simulink library "BEML_EMU_TractionInput_Lib"  (R2019b)
settings: Solver=VariableStepAuto  StartTime=0.0  StopTime=10.0  RelTol=1e-3
undefined symbols (not defined in the file): Bogie, BogieIsolationStatus, BogieSupportedMass, ContactorsFailure, DynamicBrakeForceVariation, Dynamics, ElectricalSystem, ForwardTW, HeavyWheelSlide, HeavyWheelSlip, NoEmergencyBrakeActiveTW, PowerAvailable, ReverseTW, TCMS, TCMSDynamicBrakingInhibit, TCMSEDBrakingCmd, TCMSTractionCmd, TCMSTractionInhibit, TCUPower, TractionActiveTW, TractionAuthorisation, TractionCutoff, TractionForceVariation, TractionSampleTime, TractiveLosses, VCBState, Velocity, WheelSlide, WheelSlip, WheelSpeed
libraries: simulink x4
settings Model: Creator=rleighton  LastModifiedBy=hinganes
settings DebuggingCC: ArithmeticOperatorsInVariantConditions=warning
settings SFSimCC: SimUseLocalCustomCode=off  CustomCodeUndefinedFunction=UseInterfaceOnly
settings RTWCC: RTWUseLocalCustomCode=off

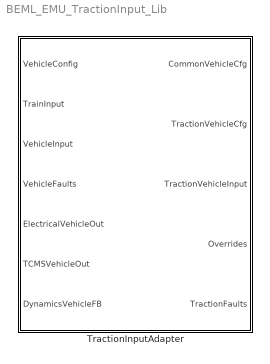
== system BEML_EMU_TractionInput_Lib ==
  TractionInputAdapter : Subsystem  TreatAsAtomicUnit=on  SystemSampleTime=TractionSampleTime

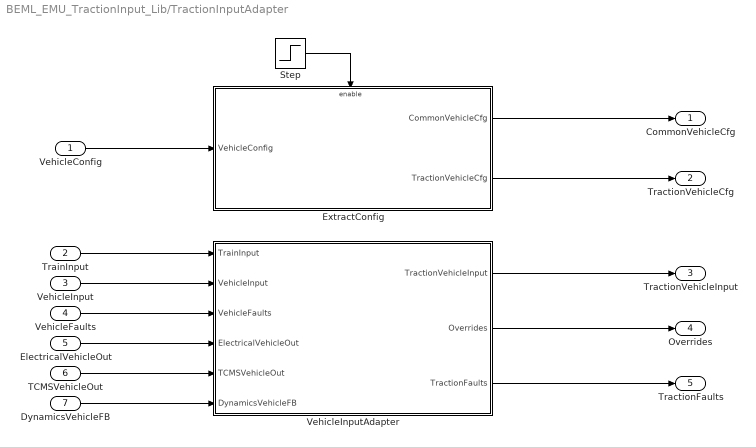
== system BEML_EMU_TractionInput_Lib/TractionInputAdapter ==
  VehicleConfig : Inport
  TrainInput : Inport  Port=2
  VehicleInput : Inport  Port=3
  VehicleFaults : Inport  Port=4
  ElectricalVehicleOut : Inport  Port=5
  TCMSVehicleOut : Inport  Port=6
  DynamicsVehicleFB : Inport  Port=7
  ExtractConfig : Subsystem
  Step : Step  Before=1  After=0
  VehicleInputAdapter : Subsystem
  CommonVehicleCfg : Outport  VectorParamsAs1DForOutWhenUnconnected=off
  TractionVehicleCfg : Outport  Port=2  VectorParamsAs1DForOutWhenUnconnected=off
  TractionVehicleInput : Outport  Port=3  VectorParamsAs1DForOutWhenUnconnected=off
  Overrides : Outport  Port=4  VectorParamsAs1DForOutWhenUnconnected=off
  TractionFaults : Outport  Port=5  VectorParamsAs1DForOutWhenUnconnected=off
  wires:
  TCMSVehicleOut/1 -> VehicleInputAdapter/5(TCMSVehicleOut)
  VehicleInputAdapter/3(TractionFaults) -> TractionFaults/1
  VehicleInputAdapter/2(Overrides) -> Overrides/1
  VehicleInputAdapter/1(TractionVehicleInput) -> TractionVehicleInput/1
  VehicleFaults/1 -> VehicleInputAdapter/3(VehicleFaults)
  Step/1 -> ExtractConfig/Enable
  ExtractConfig/2(TractionVehicleCfg) -> TractionVehicleCfg/1
  ExtractConfig/1(CommonVehicleCfg) -> CommonVehicleCfg/1
  VehicleConfig/1 -> ExtractConfig/1(VehicleConfig)
  DynamicsVehicleFB/1 -> VehicleInputAdapter/6(DynamicsVehicleFB)
  ElectricalVehicleOut/1 -> VehicleInputAdapter/4(ElectricalVehicleOut)
  VehicleInput/1 -> VehicleInputAdapter/2(VehicleInput)
  TrainInput/1 -> VehicleInputAdapter/1(TrainInput)

== system BEML_EMU_TractionInput_Lib/TractionInputAdapter/ExtractConfig ==
  VehicleConfig : Inport
  Enable : EnablePort
  ExtractConfig : Subsystem
  CommonVehicleCfg : Outport  VectorParamsAs1DForOutWhenUnconnected=off
  TractionVehicleCfg : Outport  Port=2  VectorParamsAs1DForOutWhenUnconnected=off
  wires:
  VehicleConfig/1 -> ExtractConfig/1(VehicleConfig)
  ExtractConfig/1(CommonVehicleConfig) -> CommonVehicleCfg/1
  ExtractConfig/2(TractionVehicleConfig) -> TractionVehicleCfg/1

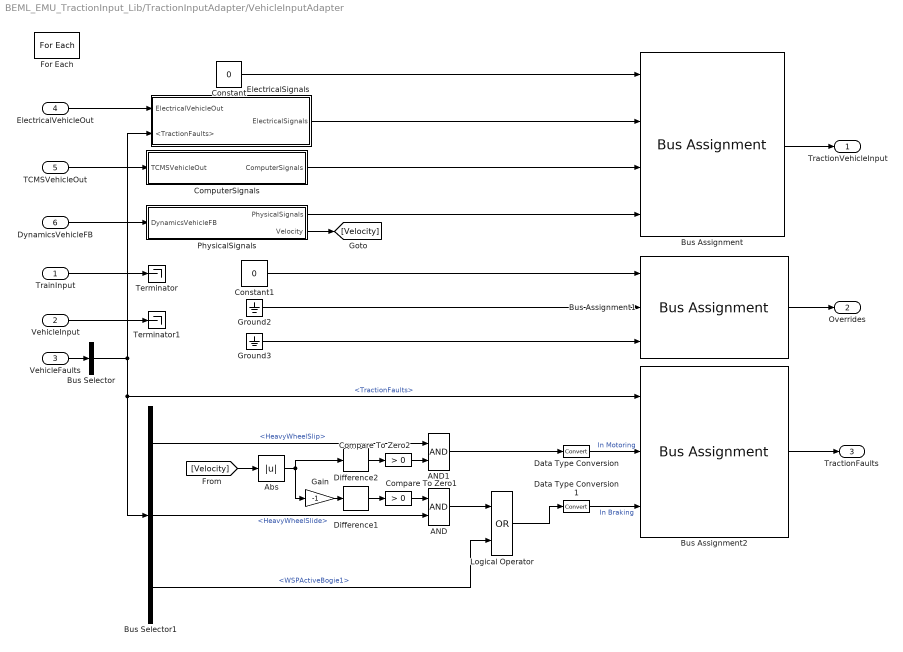
== system BEML_EMU_TractionInput_Lib/TractionInputAdapter/VehicleInputAdapter ==
  TrainInput : Inport
  VehicleInput : Inport  Port=2
  VehicleFaults : Inport  Port=3  Partition=on  PartitionDimension=1  PartitionWidth=1  PartitionOffset=0
  ElectricalVehicleOut : Inport  Port=4  Partition=on  PartitionDimension=1  PartitionWidth=1  PartitionOffset=0
  TCMSVehicleOut : Inport  Port=5  Partition=on  PartitionDimension=1  PartitionWidth=1  PartitionOffset=0
  DynamicsVehicleFB : Inport  Port=6  Partition=on  PartitionDimension=1  PartitionWidth=1  PartitionOffset=0
  AND : Logic  AllPortsSameDT=off  OutDataTypeStr=boolean
  AND1 : Logic  AllPortsSameDT=off  OutDataTypeStr=boolean
  Abs : Abs
  Bus Assignment : BusAssignment  AssignedSignals=ElectricalSystem,TCMS,Dynamics
  Bus Assignment1 : BusAssignment  AssignedSignals=TractionForceVariation,DynamicBrakeForceVariation
  Bus Assignment2 : BusAssignment  AssignedSignals=HeavyWheelSlip,HeavyWheelSlide
  Bus Selector : BusSelector  OutputSignals=TractionFaults
  Bus Selector1 : BusSelector  OutputSignals=HeavyWheelSlip,HeavyWheelSlide,WSPActiveBogie1
  Compare To Zero1 : simulink/Logic and Bit Operations/Compare To Zero  relop=>  OutDataTypeStr=boolean
  Compare To Zero2 : simulink/Logic and Bit Operations/Compare To Zero  relop=>  OutDataTypeStr=boolean
  ComputerSignals : Subsystem
  Constant : Constant  Value=0  OutDataTypeStr=Bus: BD_TractionSystem_In_Vehicle
  Constant1 : Constant  Value=0  OutDataTypeStr=Bus: BD_TractionSystem_In_Overrides
  Data Type Conversion : DataTypeConversion
  Data Type Conversion1 : DataTypeConversion
  Difference1 : simulink/Discrete/Difference  ICPrevInput=0.0  OutMin=[]  OutMax=[]  OutDataType=fixdt(1, 16)  OutScaling=2^-10  DoSatur=off
  Difference2 : simulink/Discrete/Difference  ICPrevInput=0.0  OutMin=[]  OutMax=[]  OutDataType=fixdt(1, 16)  OutScaling=2^-10  DoSatur=off
  ElectricalSignals : Subsystem
  For Each : ForEach  DisableCoverage=on
  Gain : Gain  Gain=-1
  Ground2 : Ground
  Ground3 : Ground
  Logical Operator : Logic  Operator=OR  AllPortsSameDT=off  OutDataTypeStr=boolean
  PhysicalSignals : Subsystem
  Terminator : Terminator
  Terminator1 : Terminator
  TractionVehicleInput : Outport  ConcatenationDimension=1  VectorParamsAs1DForOutWhenUnconnected=off
  Overrides : Outport  Port=2  ConcatenationDimension=1  VectorParamsAs1DForOutWhenUnconnected=off
  TractionFaults : Outport  Port=3  ConcatenationDimension=1  VectorParamsAs1DForOutWhenUnconnected=off
  wires:
  Logical Operator/1 -> Data Type Conversion1/1
  Bus Selector1/3 -> Logical Operator/2  "<WSPActiveBogie1>"
  VehicleInput/1 -> Terminator1/1
  Abs/1 -> Gain/1, Difference2/1
  Data Type Conversion1/1 -> Bus Assignment2/3  "In Braking"
  Data Type Conversion/1 -> Bus Assignment2/2  "In Motoring"
  AND/1 -> Logical Operator/1
  AND1/1 -> Data Type Conversion/1
  Compare To Zero2/1 -> AND1/2
  Difference2/1 -> Compare To Zero2/1
  [Velocity] -> Abs/1
  Bus Selector1/1 -> AND1/1  "<HeavyWheelSlip>"
  Bus Selector1/2 -> AND/2  "<HeavyWheelSlide>"
  PhysicalSignals/2(Velocity) -> [Velocity]
  Gain/1 -> Difference1/1
  Difference1/1 -> Compare To Zero1/1
  Compare To Zero1/1 -> AND/1
  Bus Assignment2/1 -> TractionFaults/1
  TCMSVehicleOut/1 -> ComputerSignals/1(TCMSVehicleOut)
  DynamicsVehicleFB/1 -> PhysicalSignals/1(DynamicsVehicleFB)
  ComputerSignals/1(ComputerSignals) -> Bus Assignment/3
  ElectricalSignals/1(ElectricalSignals) -> Bus Assignment/2
  Bus Selector/1 -> ElectricalSignals/2(<TractionFaults>), Bus Selector1/1, Bus Assignment2/1  "<TractionFaults>"
  Bus Assignment1/1 -> Overrides/1
  Ground2/1 -> Bus Assignment1/2
  Ground3/1 -> Bus Assignment1/3
  Constant1/1 -> Bus Assignment1/1
  Bus Assignment/1 -> TractionVehicleInput/1
  Constant/1 -> Bus Assignment/1
  ElectricalVehicleOut/1 -> ElectricalSignals/1(ElectricalVehicleOut)
  VehicleFaults/1 -> Bus Selector/1
  TrainInput/1 -> Terminator/1
  PhysicalSignals/1(PhysicalSignals) -> Bus Assignment/4

== system BEML_EMU_TractionInput_Lib/TractionInputAdapter/ExtractConfig/ExtractConfig ==
  VehicleConfig : Inport  Partition=on  PartitionDimension=1  PartitionWidth=1  PartitionOffset=0  BusOutputAsStruct=on
  Bus Selector : BusSelector  OutputSignals=Common,Traction
  For Each : ForEach  DisableCoverage=on
  CommonVehicleConfig : Outport  ConcatenationDimension=1  VectorParamsAs1DForOutWhenUnconnected=off
  TractionVehicleConfig : Outport  Port=2  ConcatenationDimension=1  VectorParamsAs1DForOutWhenUnconnected=off
  wires:
  Bus Selector/2 -> TractionVehicleConfig/1  "<Traction>"
  Bus Selector/1 -> CommonVehicleConfig/1  "<Common>"
  VehicleConfig/1 -> Bus Selector/1

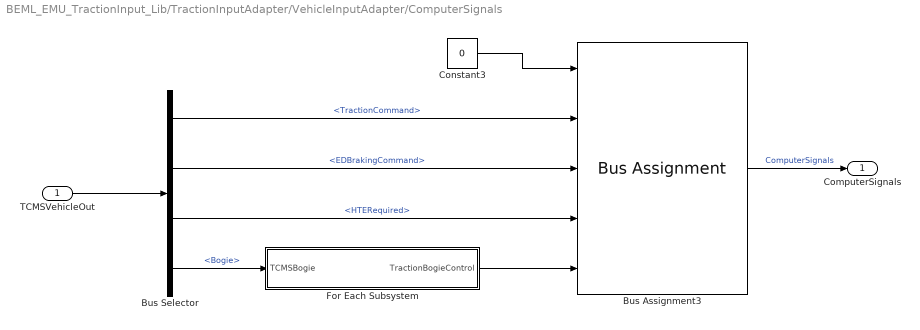
== system BEML_EMU_TractionInput_Lib/TractionInputAdapter/VehicleInputAdapter/ComputerSignals ==
  TCMSVehicleOut : Inport
  Bus Assignment3 : BusAssignment  AssignedSignals=TCMSTractionCmd,TCMSEDBrakingCmd,TractiveLosses,Bogie
  Bus Selector : BusSelector  OutputSignals=Control.TractionSBraking.TractionCommand,Control.TractionSBraking.EDBrakingCommand,Control.TractionSBraking.HTERequired,Control.TractionSBraking.Bogie
  Constant3 : Constant  Value=0  OutDataTypeStr=Bus: BD_TractionSystem_In_Vehicle_TCMS
  For Each Subsystem : Subsystem  TreatAsAtomicUnit=on
  ComputerSignals : Outport
  wires:
  Bus Selector/3 -> Bus Assignment3/4  "<HTERequired>"
  For Each Subsystem/1(TractionBogieControl) -> Bus Assignment3/5
  Bus Selector/2 -> Bus Assignment3/3  "<EDBrakingCommand>"
  Bus Selector/1 -> Bus Assignment3/2  "<TractionCommand>"
  Bus Selector/4 -> For Each Subsystem/1(TCMSBogie)  "<Bogie>"
  Constant3/1 -> Bus Assignment3/1
  Bus Assignment3/1 -> ComputerSignals/1  "ComputerSignals"
  TCMSVehicleOut/1 -> Bus Selector/1

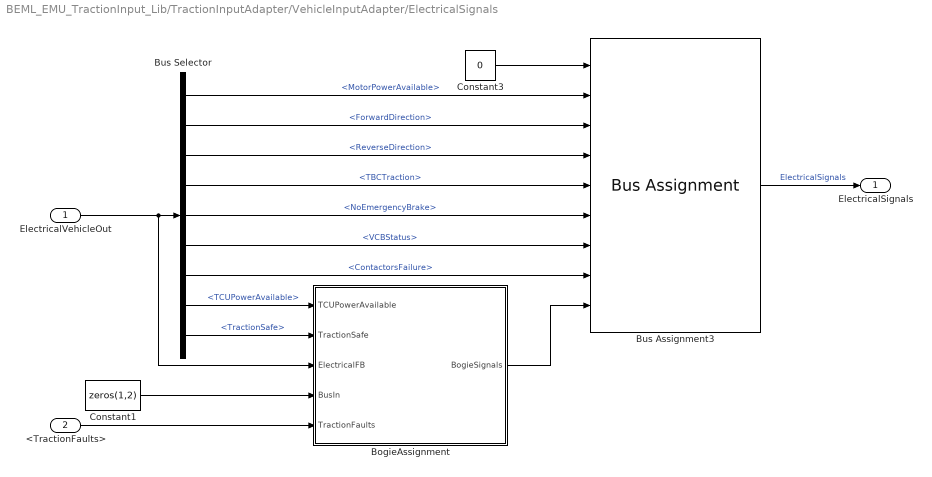
== system BEML_EMU_TractionInput_Lib/TractionInputAdapter/VehicleInputAdapter/ElectricalSignals ==
  ElectricalVehicleOut : Inport
  <TractionFaults> : Inport  Port=2
  BogieAssignment : Subsystem  TreatAsAtomicUnit=on
  Bus Assignment3 : BusAssignment  AssignedSignals=PowerAvailable,ForwardTW,ReverseTW,TractionActiveTW,NoEmergencyBrakeActiveTW,VCBState,ContactorsFailure,Bogie
  Bus Selector : BusSelector  OutputSignals=Traction.MotorPowerAvailable,Traction.ForwardDirection,Traction.ReverseDirection,Traction.TBCTraction,Traction.NoEmergencyBrake,Traction.VCBStatus,Traction.ContactorsFailure,Traction.TCUPowerAvailable,Traction.TractionSafe
  Constant1 : Constant  Value=zeros(1,2)  OutDataTypeStr=Bus: BD_TractionSystem_In_Vehicle_ElectricalSystem_Bogie
  Constant3 : Constant  Value=0  OutDataTypeStr=Bus: BD_TractionSystem_In_Vehicle_ElectricalSystem
  ElectricalSignals : Outport
  wires:
  <TractionFaults>/1 -> BogieAssignment/5(TractionFaults)
  Bus Selector/7 -> Bus Assignment3/8  "<ContactorsFailure>"
  Bus Selector/6 -> Bus Assignment3/7  "<VCBStatus>"
  BogieAssignment/1(BogieSignals) -> Bus Assignment3/9
  Bus Selector/5 -> Bus Assignment3/6  "<NoEmergencyBrake>"
  Bus Selector/8 -> BogieAssignment/1(TCUPowerAvailable)  "<TCUPowerAvailable>"
  Constant1/1 -> BogieAssignment/4(BusIn)
  Bus Selector/9 -> BogieAssignment/2(TractionSafe)  "<TractionSafe>"
  Bus Selector/4 -> Bus Assignment3/5  "<TBCTraction>"
  Bus Selector/3 -> Bus Assignment3/4  "<ReverseDirection>"
  Bus Selector/2 -> Bus Assignment3/3  "<ForwardDirection>"
  Bus Selector/1 -> Bus Assignment3/2  "<MotorPowerAvailable>"
  Constant3/1 -> Bus Assignment3/1
  Bus Assignment3/1 -> ElectricalSignals/1  "ElectricalSignals"
  ElectricalVehicleOut/1 -> Bus Selector/1, BogieAssignment/3(ElectricalFB)

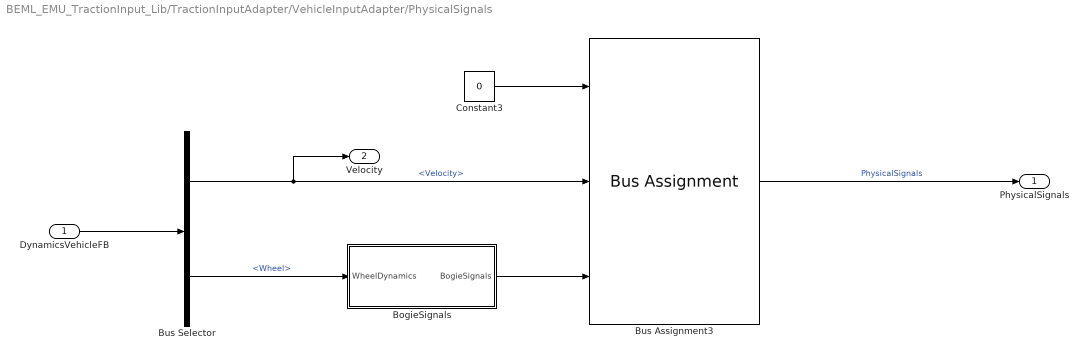
== system BEML_EMU_TractionInput_Lib/TractionInputAdapter/VehicleInputAdapter/PhysicalSignals ==
  DynamicsVehicleFB : Inport
  BogieSignals : Subsystem
  Bus Assignment3 : BusAssignment  AssignedSignals=Velocity,Bogie
  Bus Selector : BusSelector  OutputSignals=Inertia.Velocity,Wheel
  Constant3 : Constant  Value=0  OutDataTypeStr=Bus: BD_TractionSystem_In_Vehicle_Dynamics
  PhysicalSignals : Outport
  Velocity : Outport  Port=2
  wires:
  BogieSignals/1(BogieSignals) -> Bus Assignment3/3
  Bus Selector/2 -> BogieSignals/1(WheelDynamics)  "<Wheel>"
  Bus Selector/1 -> Bus Assignment3/2, Velocity/1  "<Velocity>"
  DynamicsVehicleFB/1 -> Bus Selector/1
  Bus Assignment3/1 -> PhysicalSignals/1  "PhysicalSignals"
  Constant3/1 -> Bus Assignment3/1

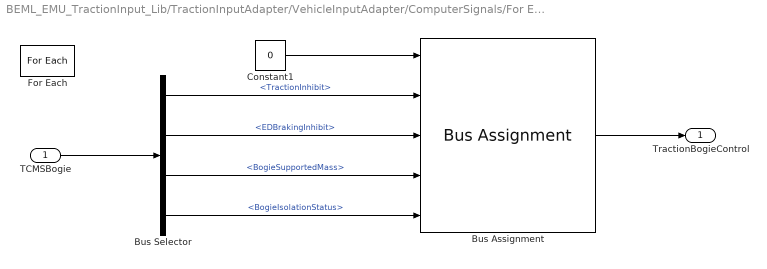
== system BEML_EMU_TractionInput_Lib/TractionInputAdapter/VehicleInputAdapter/ComputerSignals/For Each Subsystem ==
  TCMSBogie : Inport  Partition=on  PartitionDimension=1  PartitionWidth=1  PartitionOffset=0
  Bus Assignment : BusAssignment  AssignedSignals=TCMSTractionInhibit,TCMSDynamicBrakingInhibit,BogieSupportedMass,BogieIsolationStatus
  Bus Selector : BusSelector  OutputSignals=TractionInhibit,EDBrakingInhibit,BogieSupportedMass,BogieIsolationStatus
  Constant1 : Constant  Value=0  OutDataTypeStr=Bus: BD_TractionSystem_In_Vehicle_TCMS_Bogie
  For Each : ForEach  DisableCoverage=on
  TractionBogieControl : Outport  ConcatenationDimension=1
  wires:
  Bus Selector/4 -> Bus Assignment/5  "<BogieIsolationStatus>"
  Bus Selector/1 -> Bus Assignment/2  "<TractionInhibit>"
  Bus Selector/2 -> Bus Assignment/3  "<EDBrakingInhibit>"
  Bus Selector/3 -> Bus Assignment/4  "<BogieSupportedMass>"
  Bus Assignment/1 -> TractionBogieControl/1
  Constant1/1 -> Bus Assignment/1
  TCMSBogie/1 -> Bus Selector/1

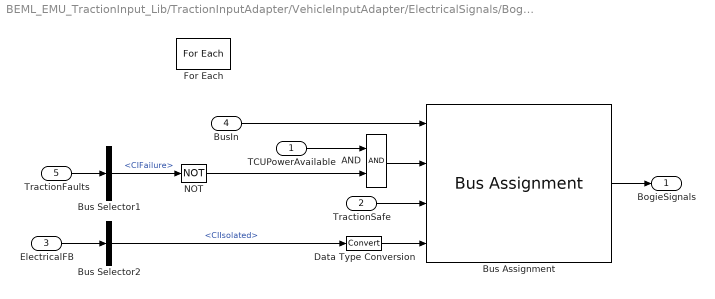
== system BEML_EMU_TractionInput_Lib/TractionInputAdapter/VehicleInputAdapter/ElectricalSignals/BogieAssignment ==
  TCUPowerAvailable : Inport
  TractionSafe : Inport  Port=2
  ElectricalFB : Inport  Port=3
  BusIn : Inport  Port=4  Partition=on  PartitionDimension=1  PartitionWidth=1  PartitionOffset=0
  TractionFaults : Inport  Port=5
  AND : Logic  AllPortsSameDT=off  OutDataTypeStr=boolean
  Bus Assignment : BusAssignment  AssignedSignals=TCUPower,TractionAuthorisation,TractionCutoff
  Bus Selector1 : BusSelector  OutputSignals=CIFailure
  Bus Selector2 : BusSelector  OutputSignals=Traction.CIIsolated
  Data Type Conversion : DataTypeConversion
  For Each : ForEach  DisableCoverage=on
  NOT : Logic  Operator=NOT  AllPortsSameDT=off  OutDataTypeStr=boolean
  BogieSignals : Outport  ConcatenationDimension=1
  wires:
  Bus Selector2/1 -> Data Type Conversion/1  "<CIIsolated>"
  ElectricalFB/1 -> Bus Selector2/1
  Data Type Conversion/1 -> Bus Assignment/4
  NOT/1 -> AND/2
  AND/1 -> Bus Assignment/2
  Bus Selector1/1 -> NOT/1  "<CIFailure>"
  TractionFaults/1 -> Bus Selector1/1
  TractionSafe/1 -> Bus Assignment/3
  TCUPowerAvailable/1 -> AND/1
  Bus Assignment/1 -> BogieSignals/1
  BusIn/1 -> Bus Assignment/1

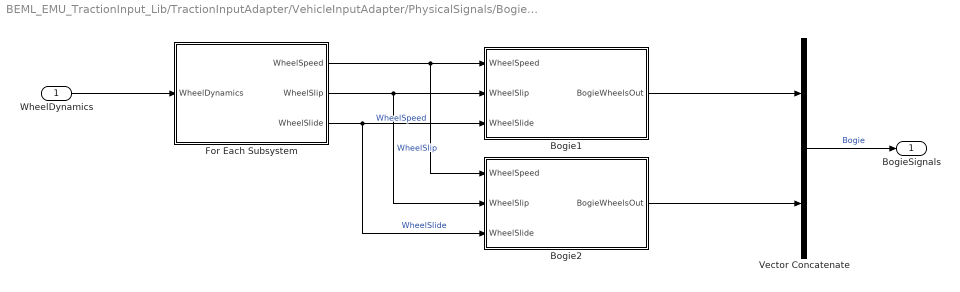
== system BEML_EMU_TractionInput_Lib/TractionInputAdapter/VehicleInputAdapter/PhysicalSignals/BogieSignals ==
  WheelDynamics : Inport
  Bogie1 : Subsystem  mask(Axle to Bogie Mapping){Indices=[1 2]}
      mask prompts: Indices "Bogie Axle Indices"
      mask help:
      | Inputs are wheel/axle-based signals of size MaxAxles (= 6)
      | Provide one-based indices of axles to be matched to bogie.
      |
      | Example: If bogie 1 has two axles, and take the two first axles outputs from dynamics, Indices vector = [1 2]
  Bogie2 : Subsystem  mask(Axle to Bogie Mapping){Indices=[3 4]}
      mask prompts: Indices "Bogie Axle Indices"
      mask help:
      | Inputs are wheel/axle-based signals of size MaxAxles (= 6)
      | Provide one-based indices of axles to be matched to bogie.
      |
      | Example: If bogie 1 has two axles, and take the two first axles outputs from dynamics, Indices vector = [1 2]
  For Each Subsystem : Subsystem  TreatAsAtomicUnit=on
  Vector Concatenate : Concatenate
  BogieSignals : Outport
  wires:
  Bogie2/1(BogieWheelsOut) -> Vector Concatenate/2
  Bogie1/1(BogieWheelsOut) -> Vector Concatenate/1
  WheelDynamics/1 -> For Each Subsystem/1(WheelDynamics)
  Vector Concatenate/1 -> BogieSignals/1  "Bogie"
  For Each Subsystem/2(WheelSlip) -> Bogie1/2(WheelSlip), Bogie2/2(WheelSlip)  "WheelSlip"
  For Each Subsystem/3(WheelSlide) -> Bogie2/3(WheelSlide), Bogie1/3(WheelSlide)  "WheelSlide"
  For Each Subsystem/1(WheelSpeed) -> Bogie1/1(WheelSpeed), Bogie2/1(WheelSpeed)  "WheelSpeed"

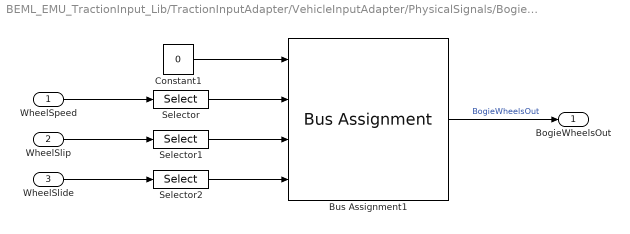
== system BEML_EMU_TractionInput_Lib/TractionInputAdapter/VehicleInputAdapter/PhysicalSignals/BogieSignals/Bogie1 ==
  WheelSpeed : Inport
  WheelSlip : Inport  Port=2
  WheelSlide : Inport  Port=3
  Bus Assignment1 : BusAssignment  AssignedSignals=WheelSpeed,WheelSlip,WheelSlide
  Constant1 : Constant  Value=0  OutDataTypeStr=Bus: BD_TractionSystem_In_Vehicle_Dynamics_Bogie
  Selector : Selector  InputPortWidth=MaxAxles  IndexOptions=Index vector (dialog)  Indices=Indices  OutputSizes=1
  Selector1 : Selector  InputPortWidth=MaxAxles  IndexOptions=Index vector (dialog)  Indices=Indices  OutputSizes=1
  Selector2 : Selector  InputPortWidth=MaxAxles  IndexOptions=Index vector (dialog)  Indices=Indices  OutputSizes=1
  BogieWheelsOut : Outport
  wires:
  Selector/1 -> Bus Assignment1/2
  WheelSlip/1 -> Selector1/1
  WheelSlide/1 -> Selector2/1
  WheelSpeed/1 -> Selector/1
  Bus Assignment1/1 -> BogieWheelsOut/1  "BogieWheelsOut"
  Selector2/1 -> Bus Assignment1/4
  Selector1/1 -> Bus Assignment1/3
  Constant1/1 -> Bus Assignment1/1

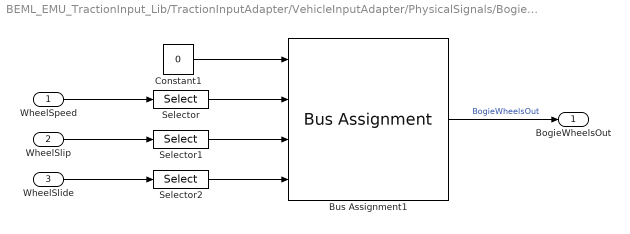
== system BEML_EMU_TractionInput_Lib/TractionInputAdapter/VehicleInputAdapter/PhysicalSignals/BogieSignals/Bogie2 ==
  WheelSpeed : Inport
  WheelSlip : Inport  Port=2
  WheelSlide : Inport  Port=3
  Bus Assignment1 : BusAssignment  AssignedSignals=WheelSpeed,WheelSlip,WheelSlide
  Constant1 : Constant  Value=0  OutDataTypeStr=Bus: BD_TractionSystem_In_Vehicle_Dynamics_Bogie
  Selector : Selector  InputPortWidth=MaxAxles  IndexOptions=Index vector (dialog)  Indices=Indices  OutputSizes=1
  Selector1 : Selector  InputPortWidth=MaxAxles  IndexOptions=Index vector (dialog)  Indices=Indices  OutputSizes=1
  Selector2 : Selector  InputPortWidth=MaxAxles  IndexOptions=Index vector (dialog)  Indices=Indices  OutputSizes=1
  BogieWheelsOut : Outport
  wires:
  Constant1/1 -> Bus Assignment1/1
  Selector1/1 -> Bus Assignment1/3
  Selector2/1 -> Bus Assignment1/4
  Bus Assignment1/1 -> BogieWheelsOut/1  "BogieWheelsOut"
  WheelSpeed/1 -> Selector/1
  WheelSlide/1 -> Selector2/1
  WheelSlip/1 -> Selector1/1
  Selector/1 -> Bus Assignment1/2

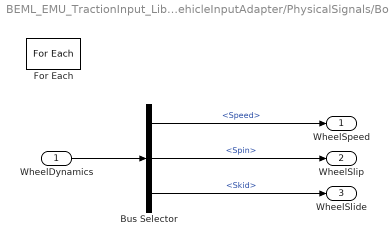
== system BEML_EMU_TractionInput_Lib/TractionInputAdapter/VehicleInputAdapter/PhysicalSignals/BogieSignals/For Each Subsystem ==
  WheelDynamics : Inport  Partition=on  PartitionDimension=1  PartitionWidth=1  PartitionOffset=0
  Bus Selector : BusSelector  OutputSignals=Speed,Spin,Skid
  For Each : ForEach  DisableCoverage=on
  WheelSpeed : Outport  ConcatenationDimension=1
  WheelSlip : Outport  Port=2  ConcatenationDimension=1
  WheelSlide : Outport  Port=3  ConcatenationDimension=1
  wires:
  Bus Selector/3 -> WheelSlide/1  "<Skid>"
  Bus Selector/2 -> WheelSlip/1  "<Spin>"
  Bus Selector/1 -> WheelSpeed/1  "<Speed>"
  WheelDynamics/1 -> Bus Selector/1
